simulink model "Adaptive_CT_ur10"  (R2022a)
settings: Solver=ode4  StartTime=0.0  StopTime=15.0  FixedStep=1e-3  RelTol=1e-5
values from neighbouring files (symbols this model uses):
  Kp = 28*diag([14 14 17 10 22 22])    [GuadagniControllore.m]
  Kv = 32*diag([14 14 17 10 22 22])    [GuadagniControllore.m]
undefined symbols (not defined in the file or in its folder): l1, l2, l3, l4, l5, l6, m1, m2, m3, m4, m5, m6, q0, r
libraries: roblocks x3
(part 1 of 9)
settings Model: Creator=pierg  LastModifiedBy=vince
settings DebuggingCC: UnconnectedInputMsg=warning  UnconnectedOutputMsg=warning  UnconnectedLineMsg=warning
settings ModelReferenceCC: ModelReferenceMinAlgLoopOccurrences=on
settings RTWCC: DLArmComputeVersion=19.05

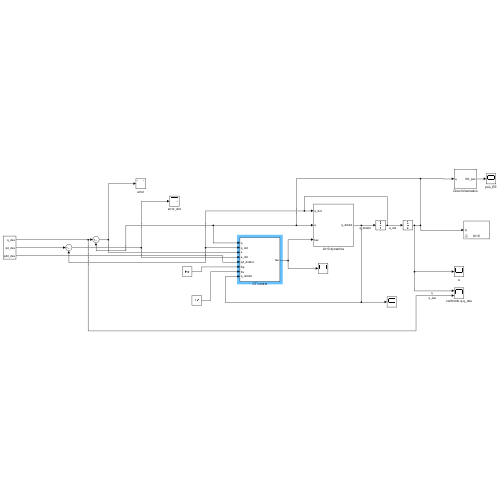
[thumbnail: Simulink's stored preview of the top-level diagram]
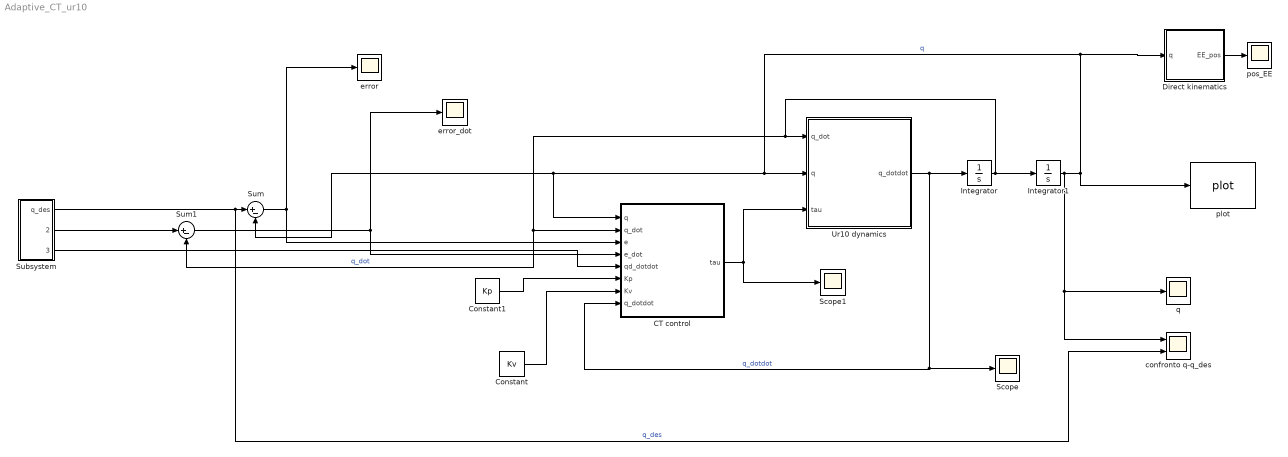
== system Adaptive_CT_ur10 ==
  CT control : Subsystem
  Constant : Constant  Value=Kv
  Constant1 : Constant  Value=Kp
  Direct kinematics : Subsystem
  Integrator : Integrator  InitialCondition=[0 0 0 0 0 0]'
  Integrator1 : Integrator  InitialCondition=q0'
  Scope : Scope
  Scope1 : Scope
  Subsystem : Subsystem
  Sum : Sum  Inputs=|+-
  Sum1 : Sum  Inputs=|+-
  Ur10 dynamics : Subsystem
  confronto q-q_des : Scope  NumInputPorts=2
  error : Scope
  error_dot : Scope
  plot : roblocks/Arm/plot  robot=ur10  fps=20  holdplot=on
  pos_EE : Scope
  q : Scope
  wires:
  Ur10 dynamics/1(q_dotdot) -> CT control/8(q_dotdot), Scope/1, Integrator/1  "q_dotdot"
  Integrator/1 -> Integrator1/1, Sum1/2, CT control/2(q_dot), Ur10 dynamics/1(q_dot)  "q_dot"
  Integrator1/1 -> confronto q-q_des/1, q/1, plot/1, Direct kinematics/1(q), Sum/2, CT control/1(q), Ur10 dynamics/2(q)  "q"
  Constant1/1 -> CT control/6(Kp)
  Constant/1 -> CT control/7(Kv)
  Subsystem/1(q_des) -> confronto q-q_des/2, Sum/1  "q_des"
  Subsystem/2(qd_des) -> Sum1/1
  Sum/1 -> CT control/3(e), error/1
  Sum1/1 -> error_dot/1, CT control/4(e_dot)
  Subsystem/3(qdd_des) -> CT control/5(qd_dotdot)
  Direct kinematics/1(EE_pos) -> pos_EE/1
  CT control/1(tau) -> Scope1/1, Ur10 dynamics/3(tau)

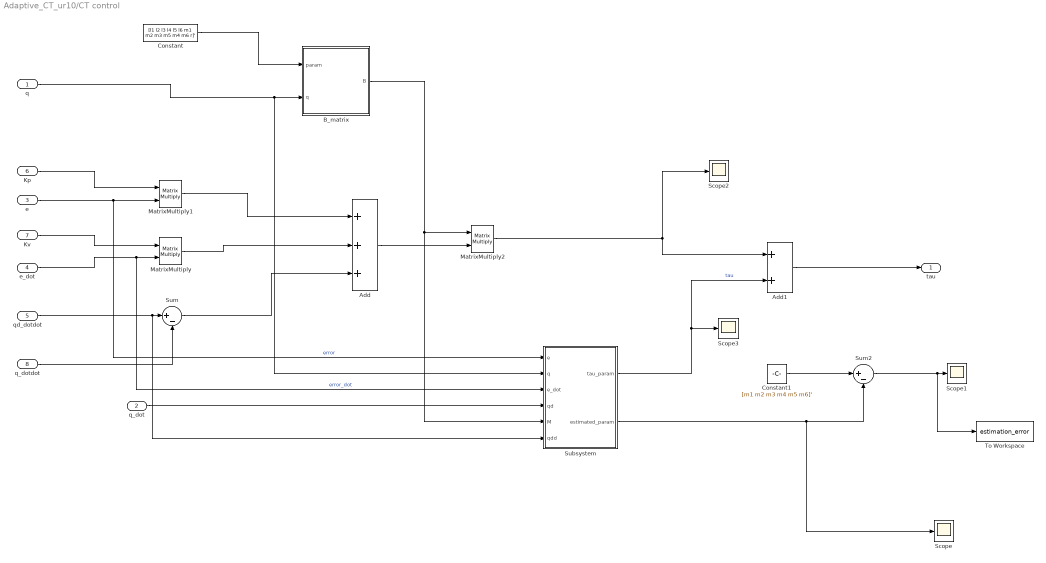
== system Adaptive_CT_ur10/CT control ==
  q : Inport
  q_dot : Inport  Port=2
  e : Inport  Port=3
  e_dot : Inport  Port=4
  qd_dotdot : Inport  Port=5
  Kp : Inport  Port=6
  Kv : Inport  Port=7
  q_dotdot : Inport  Port=8
  Add : Sum  Inputs=+++
  Add1 : Sum
  B_matrix : MATLAB Function  TreatAsAtomicUnit=on
  Constant : Constant  Value=[l1 l2 l3 l4 l5 l6 m1 m2 m3 m5 m4 m6 r]'
  Constant1 : Constant  Value=[m1 m2 m3 m4 m5 m6]'
  MatrixMultiply : Product  Multiplication=Matrix(*)
  MatrixMultiply1 : Product  Multiplication=Matrix(*)
  MatrixMultiply2 : Product  Multiplication=Matrix(*)
  Scope{,1..3} (4 alike) : Scope
  Subsystem : Subsystem
  Sum : Sum  Inputs=|+-
  Sum2 : Sum  Inputs=|+-
  To Workspace : ToWorkspace  VariableName=estimation_error  SaveFormat=Structure  SampleTime=-1
  tau : Outport
  wires:
  Subsystem/2(estimated_param) -> Sum2/2, Scope/1
  Constant/1 -> B_matrix/1(param)
  q/1 -> B_matrix/2(q), Subsystem/2(q)
  e_dot/1 -> MatrixMultiply/2, Subsystem/3(e_dot)  "error_dot"
  Kv/1 -> MatrixMultiply/1
  e/1 -> MatrixMultiply1/2, Subsystem/1(e)  "error"
  Kp/1 -> MatrixMultiply1/1
  qd_dotdot/1 -> Subsystem/6(qdd), Sum/1
  q_dotdot/1 -> Sum/2
  MatrixMultiply/1 -> Add/2
  MatrixMultiply1/1 -> Add/1
  Sum/1 -> Add/3
  Add/1 -> MatrixMultiply2/2
  B_matrix/1(B) -> MatrixMultiply2/1, Subsystem/5(M)
  q_dot/1 -> Subsystem/4(qd)
  Add1/1 -> tau/1
  Subsystem/1(tau_param) -> Scope3/1, Add1/2  "tau"
  MatrixMultiply2/1 -> Scope2/1, Add1/1
  Constant1/1 -> Sum2/1
  Sum2/1 -> To Workspace/1, Scope1/1

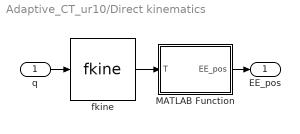
== system Adaptive_CT_ur10/Direct kinematics ==
  q : Inport
  MATLAB Function : MATLAB Function  TreatAsAtomicUnit=on
  fkine : roblocks/Arm/fkine  robot=ur10
  EE_pos : Outport
  wires:
  q/1 -> fkine/1
  MATLAB Function/1(EE_pos) -> EE_pos/1
  fkine/1 -> MATLAB Function/1(T)

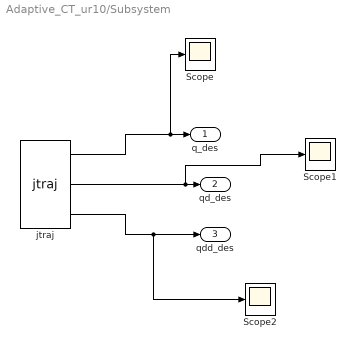
== system Adaptive_CT_ur10/Subsystem ==
  Scope : Scope
  Scope1 : Scope
  Scope2 : Scope
  jtraj : roblocks/Toolbox/jtraj  q0=q0  qf=q_des_fin  tmax=15  ts=0.01
  q_des : Outport
  qd_des : Outport  Port=2
  qdd_des : Outport  Port=3
  wires:
  jtraj/2 -> Scope1/1, qd_des/1
  jtraj/3 -> Scope2/1, qdd_des/1
  jtraj/1 -> Scope/1, q_des/1

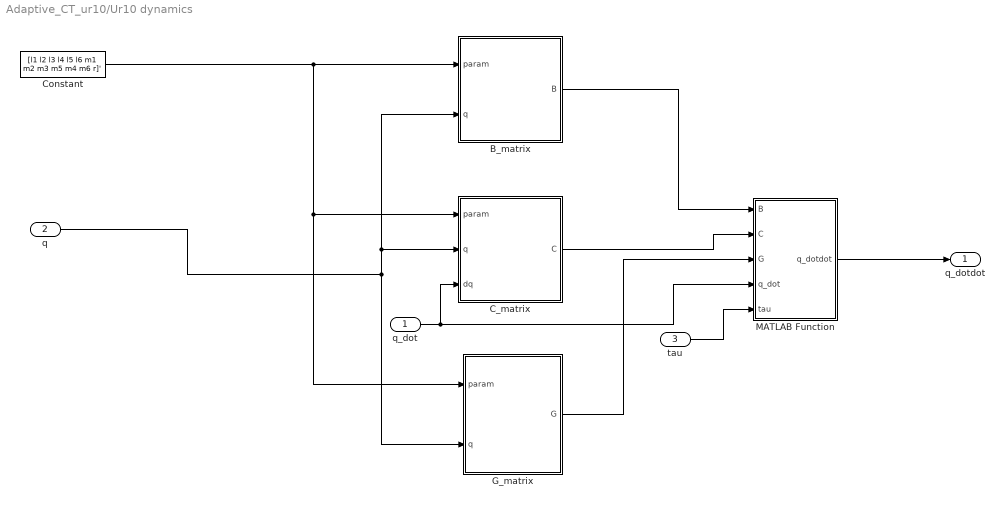
== system Adaptive_CT_ur10/Ur10 dynamics ==
  q_dot : Inport
  q : Inport  Port=2
  tau : Inport  Port=3
  B_matrix : MATLAB Function  TreatAsAtomicUnit=on
  C_matrix : MATLAB Function  TreatAsAtomicUnit=on
  Constant : Constant  Value=[l1 l2 l3 l4 l5 l6 m1 m2 m3 m5 m4 m6 r]'
  G_matrix : MATLAB Function  TreatAsAtomicUnit=on
  MATLAB Function : MATLAB Function  TreatAsAtomicUnit=on
  q_dotdot : Outport
  wires:
  Constant/1 -> G_matrix/1(param), C_matrix/1(param), B_matrix/1(param)
  q/1 -> B_matrix/2(q), C_matrix/2(q), G_matrix/2(q)
  MATLAB Function/1(q_dotdot) -> q_dotdot/1
  C_matrix/1(C) -> MATLAB Function/2(C)
  B_matrix/1(B) -> MATLAB Function/1(B)
  G_matrix/1(G) -> MATLAB Function/3(G)
  q_dot/1 -> MATLAB Function/4(q_dot), C_matrix/3(dq)
  tau/1 -> MATLAB Function/5(tau)

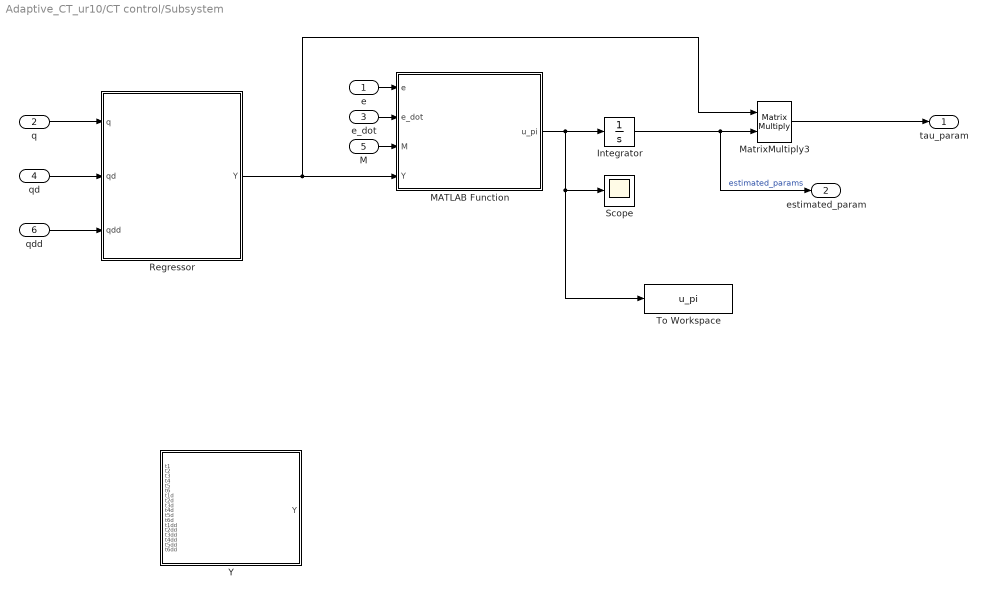
== system Adaptive_CT_ur10/CT control/Subsystem ==
  e : Inport
  q : Inport  Port=2
  e_dot : Inport  Port=3
  qd : Inport  Port=4
  M : Inport  Port=5
  qdd : Inport  Port=6
  Integrator : Integrator  InitialCondition=1.5*[m1 m2 m3 m4 m5 m6]'
  MATLAB Function : MATLAB Function  TreatAsAtomicUnit=on
  MatrixMultiply3 : Product  Multiplication=Matrix(*)
  Regressor : MATLAB Function  TreatAsAtomicUnit=on
  Scope : Scope
  To Workspace : ToWorkspace  VariableName=u_pi  SaveFormat=Structure  SampleTime=-1
  Y : MATLAB Function  TreatAsAtomicUnit=on
  tau_param : Outport
  estimated_param : Outport  Port=2
  wires:
  qd/1 -> Regressor/2(qd)
  q/1 -> Regressor/1(q)
  e_dot/1 -> MATLAB Function/2(e_dot)
  qdd/1 -> Regressor/3(qdd)
  Integrator/1 -> MatrixMultiply3/2, estimated_param/1  "estimated_params"
  e/1 -> MATLAB Function/1(e)
  M/1 -> MATLAB Function/3(M)
  Regressor/1(Y) -> MATLAB Function/4(Y), MatrixMultiply3/1
  MatrixMultiply3/1 -> tau_param/1
  MATLAB Function/1(u_pi) -> To Workspace/1, Scope/1, Integrator/1
